simulink model "modelsimulationHW"  (R2019a)
settings: Solver=FixedStepAuto  StartTime=0.0  StopTime=40.0  FixedStep=0.01  RelTol=1e-3
values from neighbouring files (symbols this model uses):
  a = 2    [ssdyn.m]    (also in transfuncHW.m)
  b = 8    [ssdyn.m]    (also in transfuncHW.m = 5)
  c = 3    [ssdyn.m]    (also in transfuncHW.m)
  d = 5    [ssdyn.m]    (also in transfuncHW.m)
settings Model: Creator=lalit  LastModifiedBy=lalit

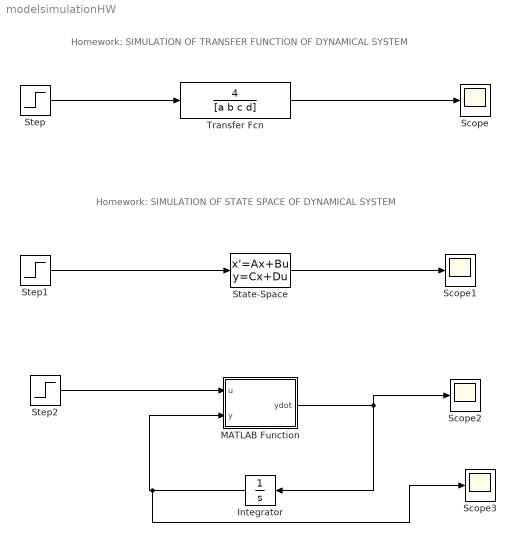
== system modelsimulationHW ==
  note: Homework: SIMULATION OF TRANSFER FUNCTION OF DYNAMICAL SYSTEM
  note: Homework: SIMULATION OF STATE SPACE OF DYNAMICAL SYSTEM
  Integrator : Integrator  InitialCondition=[0;0;0]
  MATLAB Function : MATLAB Function  TreatAsAtomicUnit=on
  Scope{,1..3} (4 alike) : Scope
  State-Space : StateSpace  A=[0 1 0; 0 0 1; -d/a -c/a -b/a]  B=[0; 0; 4/a]  C=eye(3)  D=[0; 0; 0]  InitialCondition=[0; 0; 0]
  Step : Step  Time=0  SampleTime=0
  Step1 : Step  Time=0  SampleTime=0
  Step2 : Step  Time=0  SampleTime=0
  Transfer Fcn : TransferFcn  Numerator=[4]  Denominator=[a b c d]
  wires:
  Integrator/1 -> Scope3/1, MATLAB Function/2(y)
  Step2/1 -> MATLAB Function/1(u)
  Step/1 -> Transfer Fcn/1
  MATLAB Function/1(ydot) -> Integrator/1, Scope2/1
  Step1/1 -> State-Space/1
  State-Space/1 -> Scope1/1
  Transfer Fcn/1 -> Scope/1

== matlab function modelsimulationHW/MATLAB Function ==
  data: u input; ydot output; y input
function ydot = fcn(u,y)
a=2;
b=5;
c=3;
d=5;

A=[0 1 0; 0 0 1; -d/a -c/a -b/a];
B=[0; 0; 4/a];

ydot=A*y+B*u;
